simulink subsystem "AdaptibleFIR_32taps"  (R2022a)
settings: Solver=VariableStepAuto  StartTime=0.0  StopTime=10.0  RelTol=1e-3
libraries: simulink x1
settings Model: Creator=targi  LastModifiedBy=targi

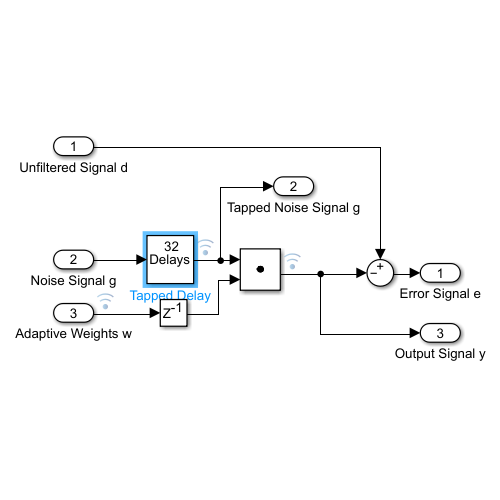
[thumbnail: Simulink's stored preview of the top-level diagram]
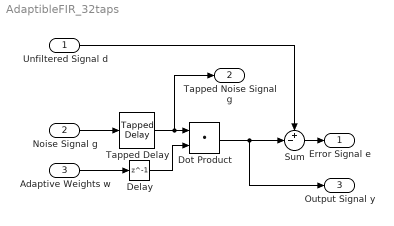
== system AdaptibleFIR_32taps ==
  Unfiltered Signal d : Inport
  Noise Signal g : Inport  Port=2
  Adaptive Weights w : Inport  Port=3
  Delay : Delay  DelayLength=1  InitialCondition=0
  Dot Product : DotProduct  OutDataTypeStr=Inherit: Inherit via internal rule
  Sum : Sum  Inputs=+-|
  Tapped Delay : simulink/Discrete/Tapped Delay  vinit=0.0  samptime=-1  NumDelays=32  DelayOrder=Newest  includeCurrent=off
  Error Signal e : Outport
  Tapped Noise Signal g : Outport  Port=2
  Output Signal y : Outport  Port=3
  wires:
  Noise Signal g/1 -> Tapped Delay/1
  Tapped Delay/1 -> Tapped Noise Signal g/1, Dot Product/1
  Dot Product/1 -> Sum/2, Output Signal y/1
  Unfiltered Signal d/1 -> Sum/1
  Sum/1 -> Error Signal e/1
  Adaptive Weights w/1 -> Delay/1
  Delay/1 -> Dot Product/2
